simulink model "spwm1"  (R2019b)
settings: Solver=VariableStepAuto  StartTime=0.0  StopTime=0.05  RelTol=1e-3
libraries: powerlib x12, simulink x2
settings Model: Creator=86153  LastModifiedBy=zou'yong
settings DataIOCC: ReturnWorkspaceOutputs=off

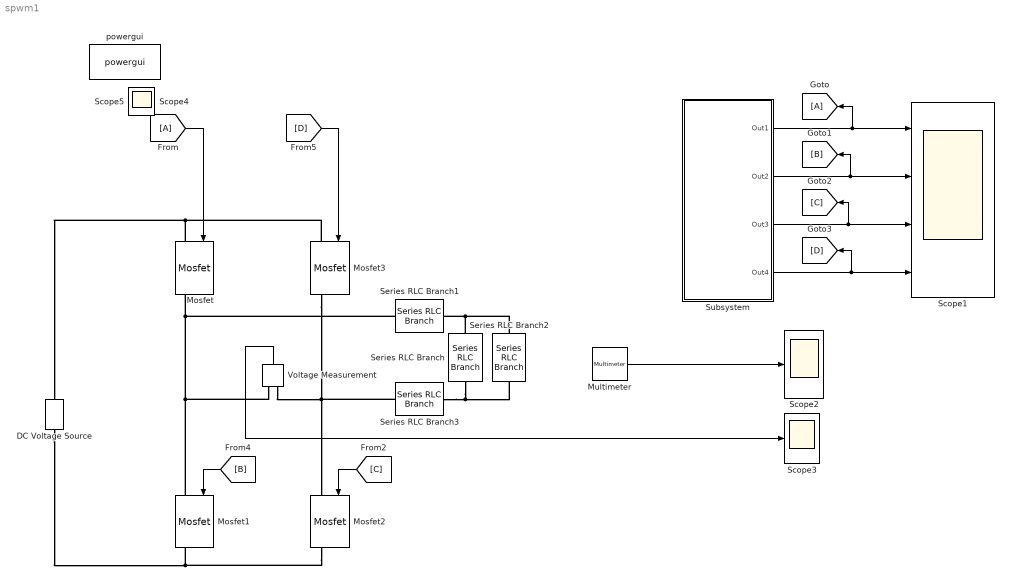
== system spwm1 ==
  DC Voltage Source : powerlib/Electrical Sources/DC Voltage Source  Amplitude=100  Measurements=None
      settings: SourceProductName=Simscape Electrical
  Mosfet{,1..3} (4 alike) : powerlib/Power Electronics/Mosfet  Ron=0.1  Lon=0  Rd=0.01  Vfd=0  IC=0  Rs=1e5  Cs=inf  Measurements=on
      settings: SourceProductName=Simscape Electrical
  Multimeter : powerlib/Measurements/Multimeter  PhasorSimulation=off  OutputType=Complex  sel=1  L=1  Gain=1  yselected={'Ub: Series RLC Branch2'};  PSBOutputType=1  PSBequivalent=0  AxesSetting=[0,0.1,-100,100]  Display=0  SavedBlockNames=-11
      settings: SourceProductName=Simscape Electrical
  Scope1 : Scope  NumInputPorts=4
  Scope{2..5} (4 alike) : Scope
  Series RLC Branch : powerlib/Elements/Series RLC Branch  LConnTagsString=__new0  RConnTagsString=__new0  BranchType=RC  Resistance=0.001  Inductance=2e-3  SetiL0=off  InitialCurrent=0  Capacitance=40e-6  Setx0=off  InitialVoltage=0  Measurements=None
      settings: SourceProductName=Simscape Electrical
  Series RLC Branch1 : powerlib/Elements/Series RLC Branch  LConnTagsString=__new0  RConnTagsString=__new0  BranchType=RL  Resistance=0.001  Inductance=2000e-6  SetiL0=off  InitialCurrent=0  Capacitance=1e-6  Setx0=off  InitialVoltage=0  Measurements=None
      settings: SourceProductName=Simscape Electrical
  Series RLC Branch2 : powerlib/Elements/Series RLC Branch  LConnTagsString=__new0  RConnTagsString=__new0  BranchType=R  Resistance=12  Inductance=2e-3  SetiL0=off  InitialCurrent=0  Capacitance=1e-6  Setx0=off  InitialVoltage=0  Measurements=Branch voltage
      settings: SourceProductName=Simscape Electrical
  Series RLC Branch3 : powerlib/Elements/Series RLC Branch  LConnTagsString=__new0  RConnTagsString=__new0  BranchType=RL  Resistance=0.001  Inductance=2000e-6  SetiL0=off  InitialCurrent=0  Capacitance=1e-6  Setx0=off  InitialVoltage=0  Measurements=None
      settings: SourceProductName=Simscape Electrical
  Subsystem : Subsystem
  Voltage Measurement : powerlib/Measurements/Voltage Measurement  PhasorSimulation=off  OutputType=Complex  PSBequivalent=0
      settings: SourceProductName=Simscape Electrical
  powergui : powerlib/powergui  Priority=1  SimulationMode=Continuous  SampleTime=50e-6  frequency=60  Iterations=50  frequencyindice=0  Pbase=100e6  ErrMax=1e-4  UnitsV=kV  UnitsW=MW  buscounter=0  FunctionMessages=off  echomessages=off  EnableUseOfTLC=off  CurrentSourceSwitches=off  DisableSnubberDevices=off  DisableRonSwitches=off  DisableVfSwitches=off  DisplayEquations=off  AutomaticDiscreteSolvers=off  SolverType=Tustin/Backward Euler (TBE)  Interpol=off  ExternalGateDelay=off  methode=off  Ts=100  x0status=blocks  SPID=on  SwTol=0  HookPort=off  NonlinearTolerance=1e-4  nMaxIteration=100  ContinueOnMaxIteration=off  RestoreLinks=warning  ResistiveCurrentMeasurement=off  Frange=[0:2:500]  Ylog=off  Xlog=on  ShowGrid=off  save=off  variable=ZData  structure=ScopeData3  ZoomFFT=off  StartTime=0  cycles=1  DisplayStyle=1  fundamental=25  FreqAxis=off  MaxFrequency=100e2  frequencyindicesteady=1  RmsSteady=1  display=off
      settings: SourceProductName=Simscape Electrical
  wires:
  [A] -> Mosfet/1
  Voltage Measurement/1 -> Scope3/1
  Subsystem/1(Out1) -> [A], Scope1/1
  Subsystem/2(Out2) -> [B], Scope1/2
  Subsystem/3(Out3) -> [C], Scope1/3
  Subsystem/4(Out4) -> [D], Scope1/4
  [B] -> Mosfet1/1
  [D] -> Mosfet3/1
  [C] -> Mosfet2/1
  Multimeter/1 -> Scope2/1
  connections:
  Mosfet1/LConn1 -- Mosfet/RConn1 -- Series RLC Branch1/RConn1 -- Voltage Measurement/LConn1
  Mosfet/LConn1 -- Mosfet3/LConn1 -- DC Voltage Source/RConn1
  DC Voltage Source/LConn1 -- Mosfet1/RConn1 -- Mosfet2/RConn1
  Series RLC Branch/LConn1 -- Series RLC Branch1/LConn1 -- Series RLC Branch2/LConn1
  Mosfet3/RConn1 -- Series RLC Branch3/RConn1 -- Mosfet2/LConn1 -- Voltage Measurement/LConn2
  Series RLC Branch/RConn1 -- Series RLC Branch3/LConn1 -- Series RLC Branch2/RConn1

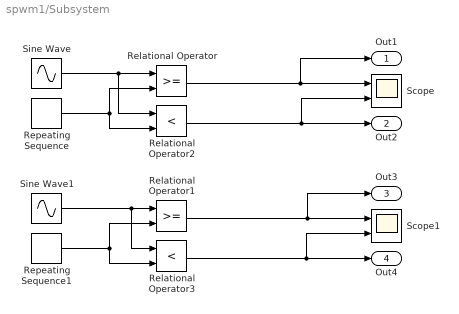
== system spwm1/Subsystem ==
  Relational Operator : RelationalOperator  OutDataTypeStr=boolean  RndMeth=Simplest
  Relational Operator1 : RelationalOperator  OutDataTypeStr=boolean  RndMeth=Simplest
  Relational Operator2 : RelationalOperator  Operator=<  OutDataTypeStr=boolean  RndMeth=Simplest
  Relational Operator3 : RelationalOperator  Operator=<  OutDataTypeStr=boolean  RndMeth=Simplest
  Repeating Sequence : simulink/Sources/Repeating Sequence  rep_seq_t=[0 1/200e3 1/100e3]  rep_seq_y=[-2 2 -2]
  Repeating Sequence1 : simulink/Sources/Repeating Sequence  rep_seq_t=[0 1/200e3 1/100e3]  rep_seq_y=[2 -2 2]
  Scope : Scope  NumInputPorts=2
  Scope1 : Scope  NumInputPorts=2
  Sine Wave : Sin  Frequency=100*pi  SampleTime=0
  Sine Wave1 : Sin  Frequency=100*pi  SampleTime=0
  Out1 : Outport
  Out2 : Outport  Port=2
  Out3 : Outport  Port=3
  Out4 : Outport  Port=4
  wires:
  Relational Operator/1 -> Out1/1, Scope/1
  Relational Operator1/1 -> Out3/1, Scope1/1
  Relational Operator2/1 -> Out2/1, Scope/2
  Relational Operator3/1 -> Out4/1, Scope1/2
  Sine Wave/1 -> Relational Operator2/1, Relational Operator/1
  Repeating Sequence/1 -> Relational Operator2/2, Relational Operator/2
  Sine Wave1/1 -> Relational Operator3/1, Relational Operator1/1
  Repeating Sequence1/1 -> Relational Operator3/2, Relational Operator1/2
